simulink model "DHN_Simulink"  (R2025a)
settings: Solver=VariableStepAuto  StartTime=0.0  StopTime=86400  RelTol=1e-3
undefined symbols (not defined in the file): mv0, x0
libraries: mpclib x1
settings Model: Creator=Muham  LastModifiedBy=Muham

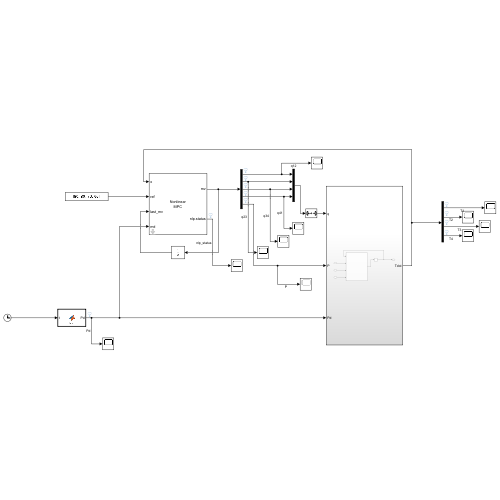
[thumbnail: Simulink's stored preview of the top-level diagram]
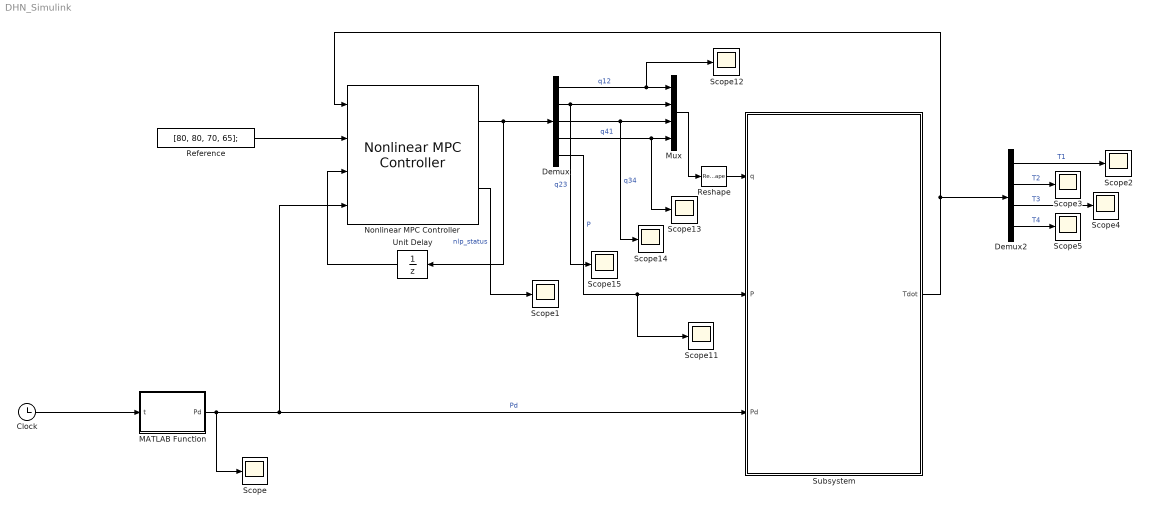
== system DHN_Simulink ==
  Clock : Clock
  Demux : Demux  Outputs=5
  Demux2 : Demux
  MATLAB Function : MATLAB Function  TreatAsAtomicUnit=on
  Mux : Mux
  Nonlinear MPC Controller : mpclib/Nonlinear MPC Controller  nlmpcobj=nlobj  UseObjectTs=on  UseMEX=off  md_enabled=on  mvtarget_enabled=off  param_enabled=off  cost_enabled=off  mvseq_enabled=off  stateseq_enabled=off  ovseq_enabled=off  slack_enabled=off  status_enabled=on  ov_min=off  ov_max=off  mv_min=off  mv_max=off  mvrate_min=off  mvrate_max=off  state_min=off  state_max=off  ov_weight=off  mv_weight=off  mvrate_weight=off  ecr_weight=off  nlp_initialize=off
  Reference : Constant  Value=[80, 80, 70, 65];  VectorParams1D=off
  Reshape : Reshape  OutputDimensionality=Row vector (2-D)
  Scope{,1..5,11..15} (11 alike) : Scope
      Scope settings: ActiveDisplayYMinimum=-1  ActiveDisplayYMaximum=1
      Scope1 settings: ActiveDisplayYMinimum=0.9  ActiveDisplayYMaximum=1.1
      Scope11 settings: ActiveDisplayYMinimum=-1  ActiveDisplayYMaximum=1  DataLoggingVariableName=ScopeData11
      Scope12 settings: ActiveDisplayYMinimum=-1  ActiveDisplayYMaximum=1  DataLoggingVariableName=ScopeData12
      Scope13 settings: ActiveDisplayYMinimum=-1  ActiveDisplayYMaximum=1  DataLoggingVariableName=ScopeData13
      Scope14 settings: ActiveDisplayYMinimum=-1  ActiveDisplayYMaximum=1  DataLoggingVariableName=ScopeData14
      Scope15 settings: ActiveDisplayYMinimum=-1  ActiveDisplayYMaximum=1  DataLoggingVariableName=ScopeData15
      Scope2 settings: ActiveDisplayYMinimum=-1  ActiveDisplayYMaximum=1  DataLoggingVariableName=ScopeData2
      Scope3 settings: ActiveDisplayYMinimum=-1  ActiveDisplayYMaximum=1  DataLoggingVariableName=ScopeData3
      Scope4 settings: ActiveDisplayYMinimum=12.980418786917747  ActiveDisplayYMaximum=70.779953468120254  DataLoggingVariableName=ScopeData4
      Scope5 settings: ActiveDisplayYMinimum=-1  ActiveDisplayYMaximum=1  DataLoggingVariableName=ScopeData5
  Subsystem : Subsystem
  Unit Delay : UnitDelay  InitialCondition=mv0  SampleTime=-1  HasFrameUpgradeWarning=on
  wires:
  Clock/1 -> MATLAB Function/1(t)
  MATLAB Function/1(Pd) -> Scope/1, Subsystem/3(Pd), Nonlinear MPC Controller/4  "Pd"
  Subsystem/1(Tdot) -> Demux2/1, Nonlinear MPC Controller/1
  Nonlinear MPC Controller/2 -> Scope1/1  "nlp_status"
  Reference/1 -> Nonlinear MPC Controller/2
  Unit Delay/1 -> Nonlinear MPC Controller/3
  Reshape/1 -> Subsystem/1(q)
  Nonlinear MPC Controller/1 -> Unit Delay/1, Demux/1
  Demux/5 -> Scope11/1, Subsystem/2(P)  "P"
  Demux/2 -> Mux/2, Scope15/1  "q23"
  Demux/1 -> Scope12/1, Mux/1  "q12"
  Demux/3 -> Scope14/1, Mux/3  "q34"
  Demux/4 -> Mux/4, Scope13/1  "q41"
  Mux/1 -> Reshape/1
  Demux2/4 -> Scope5/1  "T4"
  Demux2/3 -> Scope4/1  "T3"
  Demux2/2 -> Scope3/1  "T2"
  Demux2/1 -> Scope2/1  "T1"

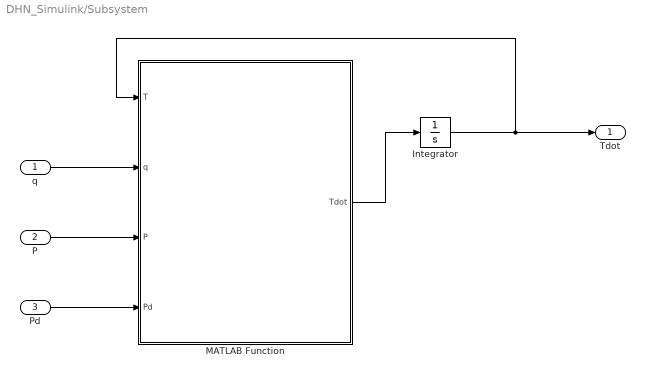
== system DHN_Simulink/Subsystem ==
  q : Inport
  P : Inport  Port=2
  Pd : Inport  Port=3
  Integrator : Integrator  InitialCondition=x0
  MATLAB Function : MATLAB Function  TreatAsAtomicUnit=on
  Tdot : Outport
  wires:
  MATLAB Function/1(Tdot) -> Integrator/1
  q/1 -> MATLAB Function/2(q)
  P/1 -> MATLAB Function/3(P)
  Pd/1 -> MATLAB Function/4(Pd)
  Integrator/1 -> MATLAB Function/1(T), Tdot/1

== matlab function DHN_Simulink/Subsystem/MATLAB Function ==
  data: Tdot output; T input; q input; P input; Pd input
function Tdot  = DHN_PlantCall(T, q, P, Pd)
%#codegen
% Wrapper for Simulink MATLAB Function block
% Calls: [Tdot, aux] = DHN_ct_plant(T, q, P, Pd)

[Tdot] = DHN_ct_plant(T, q, P, Pd);

end

== matlab function DHN_Simulink/MATLAB Function ==
  settings: updateMethod=DISCRETE
  data: t input; Pd output
function Pd = fcn(t)
% t must be simulation time in seconds
Pd = Pd_24h(t);
end
